simulink subsystem "OneActuatorFWDSSC"  (R2023a)
settings: Solver=VariableStepAuto  StartTime=0.0  StopTime=10.0  RelTol=1e-3
libraries: fl_lib x4, nesl_utility_internal x1
settings Model: Creator=The MathWorks, Inc.  LastModifiedBy=The MathWorks, Inc.
settings OptimizationCC: ReuseModelBlockBuffer=off

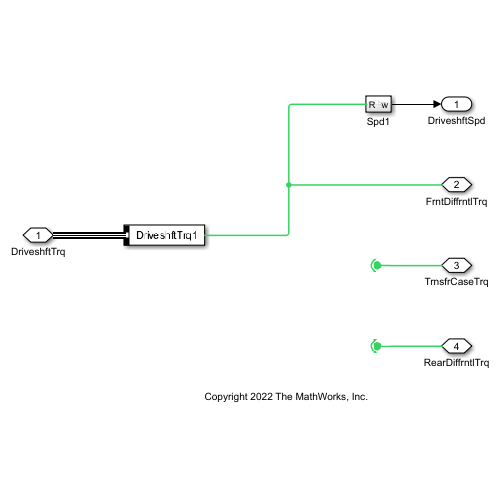
[thumbnail: Simulink's stored preview of the top-level diagram]
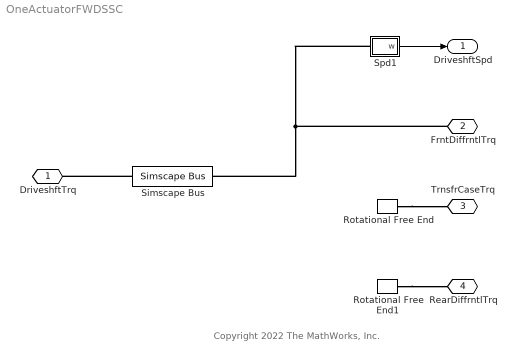
== system OneActuatorFWDSSC ==
  note: Copyright 2022 The MathWorks, Inc.
  Rotational Free End : fl_lib/Mechanical/Rotational Elements/Rotational Free End  w_specify=off  w_priority=None  w=0 rad/s  w_nominal_specify=off  w_nominal_unit=rad/s  w_nominal_value=1
      settings: SourceProductName=Foundation Library
  Rotational Free End1 : fl_lib/Mechanical/Rotational Elements/Rotational Free End  w_specify=off  w_priority=None  w=0 rad/s  w_nominal_specify=off  w_nominal_unit=rad/s  w_nominal_value=1
      settings: SourceProductName=Foundation Library
  Simscape Bus : SimscapeBus  HierarchyStrings=DriveshftTrq1
  Spd1 : Subsystem
  DriveshftTrq : PMIOPort  Side=Left
  FrntDiffrntlTrq : PMIOPort  Port=2  Side=Right
  TrnsfrCaseTrq : PMIOPort  Port=3  Side=Right
  RearDiffrntlTrq : PMIOPort  Port=4  Side=Right
  DriveshftSpd : Outport  VectorParamsAs1DForOutWhenUnconnected=off
  wires:
  Spd1/1(w) -> DriveshftSpd/1
  connections:
  FrntDiffrntlTrq/RConn1 -- Spd1/LConn1 -- Simscape Bus/LConn1
  Simscape Bus/RConn1 -- DriveshftTrq/RConn1
  Rotational Free End1/LConn1 -- RearDiffrntlTrq/RConn1
  Rotational Free End/LConn1 -- TrnsfrCaseTrq/RConn1

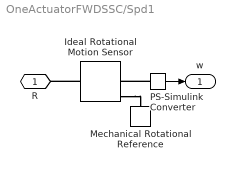
== system OneActuatorFWDSSC/Spd1 ==
  Ideal Rotational Motion Sensor : fl_lib/Mechanical/Mechanical Sensors/Ideal Rotational Motion Sensor  reference=foundation.enum.MeasurementReference.difference  acceleration_port=false  velocity_port=true  position_port=true  wrap_angle=simscape.enum.onoff.off  offset=0 rad
      settings: SourceProductName=Foundation Library
  Mechanical Rotational Reference : fl_lib/Mechanical/Rotational Elements/Mechanical Rotational Reference
      settings: SourceProductName=Foundation Library
  PS-Simulink Converter : nesl_utility_internal/PS-Simulink Converter  PhysicalDomain=network_engine_domain  SubClassName=ps_output  LeftPortType=input  RightPortType=output  PseudoPeriodic=off  Frequencies=[]  VectorFormat=inherit  Unit=inherit  AffineConversion=off
  R : PMIOPort  Side=Left
  w : Outport
  wires:
  PS-Simulink Converter/1 -> w/1
  connections:
  PS-Simulink Converter/LConn1 -- Ideal Rotational Motion Sensor/RConn2
  Ideal Rotational Motion Sensor/LConn1 -- R/RConn1
  Ideal Rotational Motion Sensor/RConn1 -- Mechanical Rotational Reference/LConn1
